simulink model "navigator"  (R2021a)
settings: Solver=FixedStepAuto  StartTime=0.0  StopTime=10.0  FixedStep=0.05  RelTol=1e-3
undefined symbols (not defined in the file): CONSTANTS_RADIUS_OF_EARTH, GF_ACTION, GF_MAX_HOR_DIST, GF_MAX_VER_DIST
(part 3 of 3)

== matlab function navigator/isBelowMaxAltitude ==
  data: home_pos input; inside_fence output; altitude input; GF_MAX_HOR_DIST parameter; GF_MAX_VER_DIST parameter; GF_ACTION parameter
function inside_fence = isBelowMaxAltitude(home_pos,altitude, GF_MAX_HOR_DIST, GF_MAX_VER_DIST, GF_ACTION)

inside_fence = true;

isHomeRequired = (GF_MAX_HOR_DIST > eps) || (GF_MAX_VER_DIST > eps) || (GF_ACTION == PX4_GEOFENCE_RESULT.GF_ACTION_RTL);
home_position_valid = (home_pos.timestamp > 0) && home_pos.valid_alt && home_pos.valid_hpos && home_pos.valid_lpos;

if isHomeRequired && home_position_valid
    dist_z = altitude - home_pos.alt;
    
    if (GF_MAX_VER_DIST > eps) && (dist_z > GF_MAX_VER_DIST)
        inside_fence = false;
    end
end

end

== matlab function navigator/isCloserThanMaxDistToHome ==
  data: home_pos input; inside_fence output; lat input; lon input; altitude input; GF_MAX_HOR_DIST parameter; GF_MAX_VER_DIST parameter; GF_ACTION parameter; CONSTANTS_RADIUS_OF_EARTH parameter
function inside_fence = isCloserThanMaxDistToHome(home_pos,lat,lon,altitude, GF_MAX_HOR_DIST, GF_MAX_VER_DIST, GF_ACTION, CONSTANTS_RADIUS_OF_EARTH)

inside_fence = true;

isHomeRequired = (GF_MAX_HOR_DIST > eps) || (GF_MAX_VER_DIST > eps) || (GF_ACTION == PX4_GEOFENCE_RESULT.GF_ACTION_RTL);
home_position_valid = (home_pos.timestamp > 0) && home_pos.valid_alt && home_pos.valid_hpos && home_pos.valid_lpos;

if isHomeRequired && home_position_valid
    [dist_xy,~,~] = get_distance_to_point_global_wgs84(lat, lon, altitude, home_pos.lat, home_pos.lon, home_pos.alt, CONSTANTS_RADIUS_OF_EARTH);
    
    if (GF_MAX_HOR_DIST > eps) && (dist_xy > GF_MAX_HOR_DIST)
        inside_fence = false;
    end
end

end
